simulink model "pendulum_with_disturbance"  (R2019a)
settings: Solver=ode45  StartTime=0.0  StopTime=50.0  MaxStep=0.01  RelTol=1e-3  EnableMultiTasking=on
values from neighbouring files (symbols this model uses):
  d = 0.2    [init_pendulum_with_disturbance.m]
  F_dist = 2.35    [init_pendulum_with_disturbance.m]
  g = 9.80665    [init_pendulum_with_disturbance.m]
  l = 1.5    [init_pendulum_with_disturbance.m]
  m = 0.5    [init_pendulum_with_disturbance.m]
  phi_0 = 0    [init_pendulum_with_disturbance.m]
  phi_dot_0 = 0    [init_pendulum_with_disturbance.m]
settings Model: Creator=TFRICKE  LastModifiedBy=MCMC
settings DataIOCC: LimitDataPoints=on  ReturnWorkspaceOutputs=off
settings OptimizationCC: LifeSpan=inf
settings DebuggingCC: SignalLabelMismatchMsg=error  BusObjectLabelMismatch=error  RootOutportRequireBusObject=error  AllowSymbolicDim=off  SFUnexpectedBacktrackingDiag=warning  SFNoUnconditionalDefaultTransitionDiag=warning  SFExecutionAtInitializationDiag=none  ArithmeticOperatorsInVariantConditions=warning
settings ModelReferenceCC: PropagateSignalLabelsOutOfModel=off
settings SFSimCC: SimUseLocalCustomCode=off
settings RTWCC: RTWUseLocalCustomCode=off
settings CodeAppCC: StateflowObjectComments=on
settings GRTTargetCC: TargetLangStandard=C89/C90 (ANSI)
settings ConfigComp: CovMetricSettings=dw  CovHtmlReporting=on  CovSaveCumulativeToWorkspaceVar=on  CovSaveSingleToWorkspaceVar=on  CovExternalEMLEnable=off

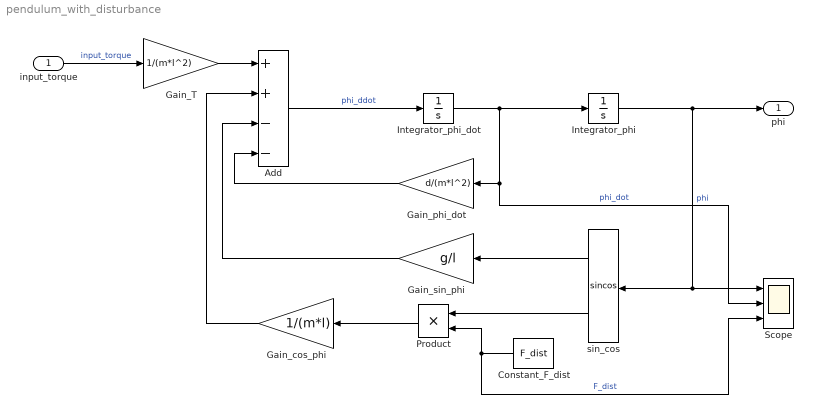
== system pendulum_with_disturbance ==
  input_torque : Inport
  Add : Sum  Inputs=++--
  Constant_F_dist : Constant  Value=F_dist
  Gain_T : Gain  Gain=1/(m*l^2)
  Gain_cos_phi : Gain  Gain=1/(m*l)
  Gain_phi_dot : Gain  Gain=d/(m*l^2)
  Gain_sin_phi : Gain  Gain=g/l
  Integrator_phi : Integrator  InitialCondition=phi_0
  Integrator_phi_dot : Integrator  InitialCondition=phi_dot_0
  Product : Product
  Scope : Scope  NumInputPorts=3
  sin_cos : Trigonometry  Operator=sincos
  phi : Outport
  wires:
  Integrator_phi_dot/1 -> Scope/2, Gain_phi_dot/1, Integrator_phi/1  "phi_dot"
  Integrator_phi/1 -> phi/1, sin_cos/1, Scope/1  "phi"
  Add/1 -> Integrator_phi_dot/1  "phi_ddot"
  sin_cos/1 -> Gain_sin_phi/1
  input_torque/1 -> Gain_T/1  "input_torque"
  sin_cos/2 -> Product/1
  Gain_phi_dot/1 -> Add/4
  Gain_sin_phi/1 -> Add/3
  Gain_cos_phi/1 -> Add/2
  Gain_T/1 -> Add/1
  Constant_F_dist/1 -> Scope/3, Product/2  "F_dist"
  Product/1 -> Gain_cos_phi/1
